simulink model "Lorenz_habr32"  (R2014a)
settings: Solver=FixedStepDiscrete  SolverMode=SingleTasking  StartTime=0.0  StopTime=30  FixedStep=0.01  RelTol=1e-3
libraries: xbsIndex_r4 x26, simulink x3
settings Model: Creator=Administrator  LastModifiedBy=Kapitanov
settings DataIOCC: SignalLoggingSaveFormat=ModelDataLogs
settings OptimizationCC: ExpressionDepthLimit=2147483647
settings DebuggingCC: UnderspecifiedInitializationDetection=Classic  FcnCallInpInsideContextMsg=UseLocalSettings  StateNameClashWarn=warning
settings GRTTargetCC: CombineOutputUpdateFcns=off  GRTInterface=on

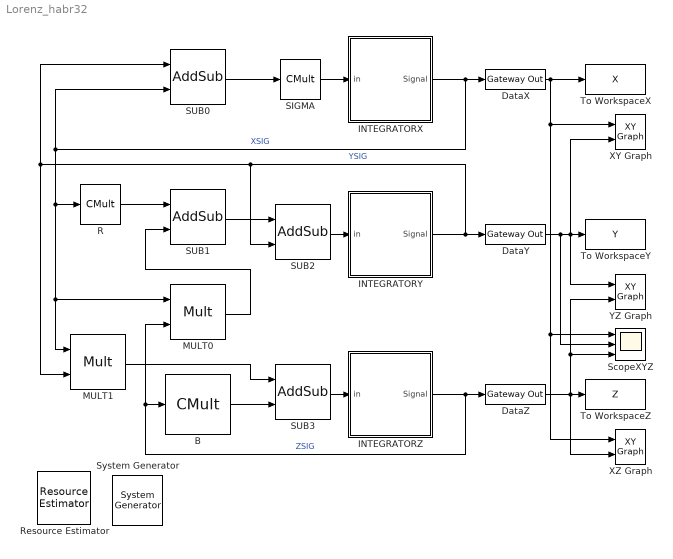
== system Lorenz_habr32 ==
  " System Generator" : xbsIndex_r4/ System Generator  Tag=genX  xilinxfamily=kintex7  part=xc7k325t  speed=-3  package=fbg676  synthesis_tool=XST  clock_wrapper=Clock Enables  directory=./netlist  proj_type=Project Navigator  Synth_file=XST Defaults  Impl_file=ISE Defaults  testbench=off  simulink_period=0.01  sysclk_period=10  dcm_input_clock_period=10  incr_netlist=off  trim_vbits=Everywhere in SubSystem  dbl_ovrd=According to Block Masks  core_generation=According to Block Masks  run_coregen=off  deprecated_control=off  eval_field=0  block_type=sysgen
  B : xbsIndex_r4/CMult  const=8/3  gui_display_data_type=Fixed-point  const_n_bits=32  const_bin_pt=12  float_type=Single  exp_bits=8  fraction_bits=24  en=off  latency=0  precision=User Defined  arith_type="Signed  (2's comp)"  n_bits=64  bin_pt=52  quantization="Round  (unbiased: +/- Inf)"  overflow=Wrap  dbl_ovrd=off  use_behavioral_HDL=off  mem_type=Distributed RAM  pipeline=off  block_type=cmult
  DataX : xbsIndex_r4/Gateway Out  inherit_from_input=off  hdl_port=on  timing_constraint=None  locs_specified=off  LOCs={}  UseAsDAC=off  DACChannel='1'  block_type=gatewayout
  DataY : xbsIndex_r4/Gateway Out  inherit_from_input=off  hdl_port=on  timing_constraint=None  locs_specified=off  LOCs={}  UseAsDAC=off  DACChannel='1'  block_type=gatewayout
  DataZ : xbsIndex_r4/Gateway Out  inherit_from_input=off  hdl_port=on  timing_constraint=None  locs_specified=off  LOCs={}  UseAsDAC=off  DACChannel='1'  block_type=gatewayout
  INTEGRATORX : Subsystem
  INTEGRATORY : Subsystem
  INTEGRATORZ : Subsystem
  MULT0 : xbsIndex_r4/Mult  precision=User Defined  arith_type="Signed  (2's comp)"  n_bits=32  bin_pt=12  quantization=Truncate  overflow=Wrap  en=off  latency=0  dbl_ovrd=off  use_behavioral_HDL=off  opt=Speed  use_embedded=on  optimum_pipeline=off  pipeline=on  use_rpm=on  placement_style=Triangular  block_type=mult
  MULT1 : xbsIndex_r4/Mult  precision=User Defined  arith_type="Signed  (2's comp)"  n_bits=32  bin_pt=12  quantization=Truncate  overflow=Wrap  en=off  latency=0  dbl_ovrd=off  use_behavioral_HDL=off  opt=Speed  use_embedded=on  optimum_pipeline=off  pipeline=on  use_rpm=on  placement_style=Triangular  block_type=mult
  R : xbsIndex_r4/CMult  const=28  gui_display_data_type=Fixed-point  const_n_bits=32  const_bin_pt=12  float_type=Single  exp_bits=8  fraction_bits=24  en=off  latency=0  precision=User Defined  arith_type="Signed  (2's comp)"  n_bits=64  bin_pt=52  quantization="Round  (unbiased: +/- Inf)"  overflow=Wrap  dbl_ovrd=off  use_behavioral_HDL=off  mem_type=Distributed RAM  pipeline=off  block_type=cmult
      settings: block_version=11.1
  Resource Estimator : xbsIndex_r4/Resource Estimator  Tag=resEstTag  Slices=100  FFs=500  BRAMs=20  LUTs=500  IOBs=48  EBMs=10  TBUFs=0  xl_use_estimator_area=off  est_options=Estimate  block_type=resource_estimator
      settings: AttributesFormatString=Resource\nEstimator
  SIGMA : xbsIndex_r4/CMult  const=10  gui_display_data_type=Fixed-point  const_n_bits=32  const_bin_pt=12  float_type=Single  exp_bits=8  fraction_bits=24  en=off  latency=0  precision=User Defined  arith_type="Signed  (2's comp)"  n_bits=64  bin_pt=52  quantization="Round  (unbiased: +/- Inf)"  overflow=Wrap  dbl_ovrd=off  use_behavioral_HDL=off  mem_type=Distributed RAM  pipeline=off  block_type=cmult
      settings: block_version=11.1
  SUB{0..3} (4 alike) : xbsIndex_r4/AddSub  mode=Subtraction  use_carryin=off  use_carryout=off  en=off  latency=0  precision=User Defined  arith_type="Signed  (2's comp)"  n_bits=32  bin_pt=12  quantization="Round  (unbiased: +/- Inf)"  overflow=Wrap  dbl_ovrd=off  use_behavioral_HDL=off  hw_selection=Fabric  pipelined=off  block_type=addsub
      settings: block_version=11.1
  ScopeXYZ : Scope  NumInputPorts=3
      settings: Description=XYZ in time  TimeRange=50  YMin=-20~-25~5  YMax=20~25~50  SampleInput=on
  To WorkspaceX : ToWorkspace  VariableName=X  SampleTime=0.01
  To WorkspaceY : ToWorkspace  VariableName=Y  SampleTime=0.01
  To WorkspaceZ : ToWorkspace  VariableName=Z  SampleTime=0.01
  XY Graph : simulink/Sinks/XY Graph  xmin=-30  xmax=30  ymin=-30  ymax=30  st=-1
  XZ Graph : simulink/Sinks/XY Graph  xmin=-30  xmax=30  ymin=0  ymax=60  st=-1
  YZ Graph : simulink/Sinks/XY Graph  xmin=-30  xmax=30  ymin=0  ymax=60  st=-1
  wires:
  SIGMA/1 -> INTEGRATORX/1(in)
  INTEGRATORX/1(Signal) -> MULT0/1, MULT1/1, R/1, SUB0/2, DataX/1  "XSIG"
  SUB0/1 -> SIGMA/1
  R/1 -> SUB1/1
  INTEGRATORY/1(Signal) -> MULT1/2, SUB0/1, SUB2/2, DataY/1  "YSIG"
  SUB1/1 -> SUB2/1
  SUB2/1 -> INTEGRATORY/1(in)
  MULT0/1 -> SUB1/2
  INTEGRATORZ/1(Signal) -> MULT0/2, B/1, DataZ/1  "ZSIG"
  SUB3/1 -> INTEGRATORZ/1(in)
  MULT1/1 -> SUB3/1
  B/1 -> SUB3/2
  DataX/1 -> XY Graph/1, ScopeXYZ/1, XZ Graph/1, To WorkspaceX/1
  DataY/1 -> XY Graph/2, To WorkspaceY/1, YZ Graph/1, ScopeXYZ/2
  DataZ/1 -> To WorkspaceZ/1, XZ Graph/2, YZ Graph/2, ScopeXYZ/3

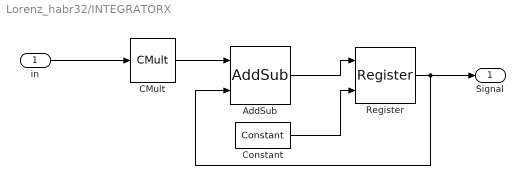
== system Lorenz_habr32/INTEGRATORX ==
  in : Inport  SampleTime=0.01
  AddSub : xbsIndex_r4/AddSub  mode=Addition  use_carryin=off  use_carryout=off  en=off  latency=0  precision=User Defined  arith_type="Signed  (2's comp)"  n_bits=32  bin_pt=12  quantization="Round  (unbiased: +/- Inf)"  overflow=Wrap  dbl_ovrd=off  use_behavioral_HDL=off  hw_selection=Fabric  pipelined=off  block_type=addsub
  CMult : xbsIndex_r4/CMult  const=1/100  gui_display_data_type=Fixed-point  const_n_bits=32  const_bin_pt=12  float_type=Single  exp_bits=8  fraction_bits=24  en=off  latency=0  precision=User Defined  arith_type="Signed  (2's comp)"  n_bits=64  bin_pt=52  quantization="Round  (unbiased: +/- Inf)"  overflow=Wrap  dbl_ovrd=off  use_behavioral_HDL=off  mem_type=Distributed RAM  pipeline=off  block_type=cmult
      settings: block_version=11.1
  Constant : xbsIndex_r4/Constant  const=0  gui_display_data_type=Fixed-point  arith_type=Boolean  n_bits=32  bin_pt=14  preci_type=Single  exp_width=8  frac_width=24  explicit_period=on  period=0.01  equ=P=C  opselect=C  inp2=PCIN>>17  opr=+  inp1=P  carry=CIN  dbl_ovrd=off  block_type=constant
      settings: block_version=11.1
  Register : xbsIndex_r4/Register  init=10  rst=on  en=off  dbl_ovrd=off  block_type=register
      settings: block_version=11.1
  Signal : Outport  SampleTime=0.01
  wires:
  AddSub/1 -> Register/1
  Register/1 -> Signal/1, AddSub/2
  CMult/1 -> AddSub/1
  in/1 -> CMult/1
  Constant/1 -> Register/2

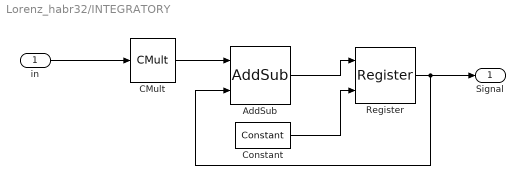
== system Lorenz_habr32/INTEGRATORY ==
  in : Inport  SampleTime=0.01
  AddSub : xbsIndex_r4/AddSub  mode=Addition  use_carryin=off  use_carryout=off  en=off  latency=0  precision=User Defined  arith_type="Signed  (2's comp)"  n_bits=32  bin_pt=12  quantization="Round  (unbiased: +/- Inf)"  overflow=Wrap  dbl_ovrd=off  use_behavioral_HDL=off  hw_selection=Fabric  pipelined=off  block_type=addsub
  CMult : xbsIndex_r4/CMult  const=1/100  gui_display_data_type=Fixed-point  const_n_bits=32  const_bin_pt=12  float_type=Single  exp_bits=8  fraction_bits=24  en=off  latency=0  precision=User Defined  arith_type="Signed  (2's comp)"  n_bits=64  bin_pt=52  quantization="Round  (unbiased: +/- Inf)"  overflow=Wrap  dbl_ovrd=off  use_behavioral_HDL=off  mem_type=Distributed RAM  pipeline=off  block_type=cmult
      settings: block_version=11.1
  Constant : xbsIndex_r4/Constant  const=0  gui_display_data_type=Fixed-point  arith_type=Boolean  n_bits=32  bin_pt=14  preci_type=Single  exp_width=8  frac_width=24  explicit_period=on  period=0.01  equ=P=C  opselect=C  inp2=PCIN>>17  opr=+  inp1=P  carry=CIN  dbl_ovrd=off  block_type=constant
      settings: block_version=11.1
  Register : xbsIndex_r4/Register  init=10  rst=on  en=off  dbl_ovrd=off  block_type=register
      settings: block_version=11.1
  Signal : Outport  SampleTime=0.01
  wires:
  AddSub/1 -> Register/1
  Register/1 -> Signal/1, AddSub/2
  CMult/1 -> AddSub/1
  in/1 -> CMult/1
  Constant/1 -> Register/2

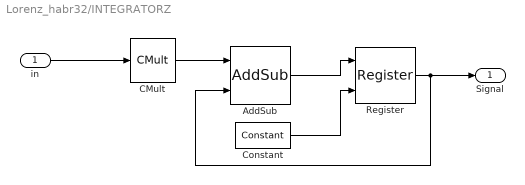
== system Lorenz_habr32/INTEGRATORZ ==
  in : Inport  SampleTime=0.01
  AddSub : xbsIndex_r4/AddSub  mode=Addition  use_carryin=off  use_carryout=off  en=off  latency=0  precision=User Defined  arith_type="Signed  (2's comp)"  n_bits=32  bin_pt=12  quantization="Round  (unbiased: +/- Inf)"  overflow=Wrap  dbl_ovrd=off  use_behavioral_HDL=off  hw_selection=Fabric  pipelined=off  block_type=addsub
  CMult : xbsIndex_r4/CMult  const=1/100  gui_display_data_type=Fixed-point  const_n_bits=32  const_bin_pt=12  float_type=Single  exp_bits=8  fraction_bits=24  en=off  latency=0  precision=User Defined  arith_type="Signed  (2's comp)"  n_bits=64  bin_pt=52  quantization="Round  (unbiased: +/- Inf)"  overflow=Wrap  dbl_ovrd=off  use_behavioral_HDL=off  mem_type=Distributed RAM  pipeline=off  block_type=cmult
      settings: block_version=11.1
  Constant : xbsIndex_r4/Constant  const=0  gui_display_data_type=Boolean  arith_type=Boolean  n_bits=32  bin_pt=14  preci_type=Single  exp_width=8  frac_width=24  explicit_period=on  period=0.01  equ=P=C  opselect=C  inp2=PCIN>>17  opr=+  inp1=P  carry=CIN  dbl_ovrd=off  block_type=constant
      settings: block_version=11.1
  Register : xbsIndex_r4/Register  init=10  rst=on  en=off  dbl_ovrd=off  block_type=register
      settings: block_version=11.1
  Signal : Outport  SampleTime=0.01
  wires:
  AddSub/1 -> Register/1
  Register/1 -> Signal/1, AddSub/2
  CMult/1 -> AddSub/1
  in/1 -> CMult/1
  Constant/1 -> Register/2
